simulink model "Control_Model"  (R2024b)
settings: Solver=FixedStepDiscrete  StartTime=0.0  StopTime=10.0  FixedStep=50e-6  MaxStep=1e-6  RelTol=1e-3
values from neighbouring files (symbols this model uses):
  Id_ki = Rs / tau    (= 1250)    [PID_Data.m]    (also in PMSM_PID_Data.m = 900)
  Id_kp = Ld / tau    (= 12.5)    [PID_Data.m]    (also in PMSM_PID_Data.m = 0.5)
  Iq_ki = Rs / tau    (= 1250)    [PID_Data.m]    (also in PMSM_PID_Data.m = 900)
  Iq_kp = Lq / tau    (= 12.5)    [PID_Data.m]    (also in PMSM_PID_Data.m = 0.5)
  Lambda = 0.175    [PID_Data.m]    (also in PMSM_PID_Data.m = (Ke_LL/sqrt(3)) / (p * 1000*2*pi/60))
  Ld = 0.005    [PID_Data.m]    (also in PMSM_PID_Data.m = 0.0002)
  lower_limit = -86.55    [PID_Data.m]    (also in PMSM_PID_Data.m = -20)
  Lq = 0.005    [PID_Data.m]    (also in PMSM_PID_Data.m = 0.0002)
  p = 4    [PID_Data.m]    (also in PMSM_PID_Data.m)
  Spd_Kb = Ki_radps    (= 47.619047619)    [PID_Data.m]    (also in PMSM_PID_Data.m = Spd_ki/Spd_kp)
  Spd_ki = Ki_radps*(2*pi/60)    (= 4.9866550057)    [PID_Data.m]    (also in PMSM_PID_Data.m = Ki_radps*(2*pi/60))
  Spd_kp = Kp_radps*(2*pi/60)    (= 0.0282045207122)    [PID_Data.m]    (also in PMSM_PID_Data.m = Kp_radps*(2*pi/60))
  Spd_lower_limit = -Iq_ref_limit    (= -10)    [PID_Data.m]    (also in PMSM_PID_Data.m = -7.1)
  Spd_upper_limit = Iq_ref_limit    (= 10)    [PID_Data.m]    (also in PMSM_PID_Data.m = 7.1)
  Ts = 1/20000    (= 5e-05)    [PID_Data.m]    (also in PMSM_PID_Data.m)
  Uabc_limit = 2/Vdc    (= 0.00666666666667)    [PID_Data.m]    (also in PMSM_PID_Data.m = 0.05)
  upper_limit = 86.55    [PID_Data.m]    (also in PMSM_PID_Data.m = 20)
  Vdc = 300    [PID_Data.m]    (also in PMSM_PID_Data.m = 40)
libraries: slpidlib x3, mcbcontrolslib x1
settings Model: Creator=BitCore  LastModifiedBy=BitCore

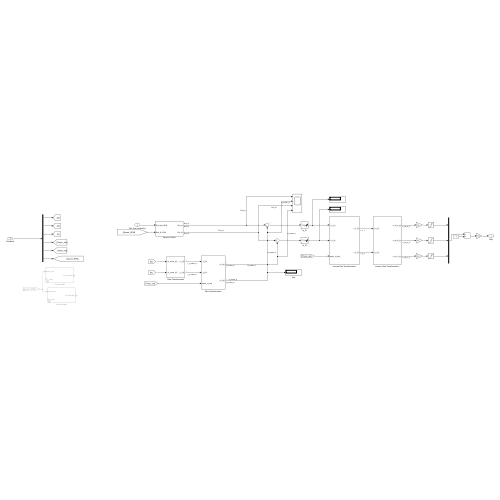
[thumbnail: Simulink's stored preview of the top-level diagram]
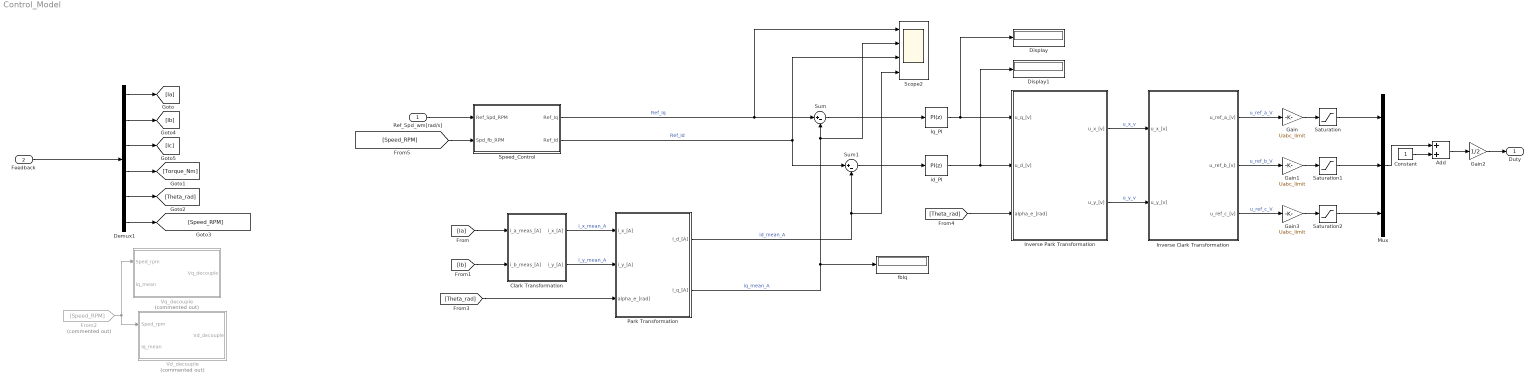
== system Control_Model ==
  Ref_Spd_wm[rad/s] : Inport
  Feedback : Inport  Port=2  OutDataTypeStr=single
  Add : Sum
  Clark Transformation : Subsystem
  Constant : Constant
  Demux1 : Demux  Outputs=6
  Display : Display
  Display1 : Display
  From2 : From  Commented=on  GotoTag=Speed_RPM
  Gain : Gain  Gain=Uabc_limit
  Gain1 : Gain  Gain=Uabc_limit
  Gain2 : Gain  Gain=1/2
  Gain3 : Gain  Gain=Uabc_limit
  "Inverse Clark Transformation " : Subsystem
  Inverse Park Transformation : Subsystem
  Iq_PI : slpidlib/PID Controller  Controller=PI  Form=Parallel  TimeDomain=Discrete-time  UseExternalTs=off  SampleTime=Ts  IntegratorMethod=Forward Euler  FilterMethod=Forward Euler  ControllerParametersSource=internal  P=Iq_kp  I=Iq_ki  UseKiTs=off  D=0  UseExternalDerivativeSource=off  N=100  UseFilter=on  TunerSelectOption=Transfer Function Based (PID Tuner App)  InitialConditionSource=internal  InitialConditionForIntegrator=0  InitialConditionForFilter=0  DifferentiatorICPrevScaledInput=0  ExternalReset=none  TrackingMode=off  Kt=1  LimitOutput=on  SatLimitsSource=internal  UpperSaturationLimit=upper_limit  LowerSaturationLimit=lower_limit  LinearizeAsGain=on  AntiWindupMode=back-calculation  Kb=1  LimitIntegrator=off  UpperIntegratorSaturationLimit=inf  LowerIntegratorSaturationLimit=-inf  POutMin=[]  POutMax=[]  IOutMin=[]  IOutMax=[]  DOutMin=[]  DOutMax=[]  NOutMin=[]  NOutMax=[]  SumOutMin=[]  SumOutMax=[]  SaturationOutMin=[]  SaturationOutMax=[]  PParamMin=[]  PParamMax=[]  IParamMin=[]  IParamMax=[]  DParamMin=[]  DParamMax=[]  NParamMin=[]  NParamMax=[]  KbParamMin=[]  KbParamMax=[]  KtParamMin=[]  KtParamMax=[]  KbOutMin=[]  KbOutMax=[]  KtOutMin=[]  KtOutMax=[]  IntegratorOutMin=[]  IntegratorOutMax=[]  FilterOutMin=[]  FilterOutMax=[]  SumI1OutMin=[]  SumI1OutMax=[]  SumI2OutMin=[]  SumI2OutMax=[]  SumI3OutMin=[]  SumI3OutMax=[]  SumI4OutMin=[]  SumI4OutMax=[]  SumDOutMin=[]  SumDOutMax=[]  DifferentiatorOutMin=[]  DifferentiatorOutMax=[]  FilterDiffOutCoefMin=[]  FilterDiffOutCoefMax=[]  ReciprocalOutMin=[]  ReciprocalOutMax=[]  SumDenOutMin=[]  SumDenOutMax=[]  SumNumOutMin=[]  SumNumOutMax=[]  DivideOutMin=[]  DivideOutMax=[]  UdiffTsProdOutMin=[]  UdiffTsProdOutMax=[]  NTsProdOutMin=[]  NTsProdOutMax=[]  UintegralTsProdOutMin=[]  UintegralTsProdOutMax=[]  UngainTsProdOutMin=[]  UngainTsProdOutMax=[]  ClampingZeroOutDataTypeStr=Inherit: Inherit via back propagation  ClampingZeroOutMin=[]  ClampingZeroOutMax=[]  FilterDenConstantOutDataTypeStr=Inherit: Inherit via back propagation  FilterDenConstantOutMin=[]  FilterDenConstantOutMax=[]  PCopyOutDataTypeStr=Inherit: Inherit via back propagation  PCopyOutMin=[]  PCopyOutMax=[]  NCopyOutDataTypeStr=Inherit: Inherit via back propagation  NCopyOutMin=[]  NCopyOutMax=[]  IntegratorContinuousStateAttributes=''  IntegratorStateMustResolveToSignalObject=off  IntegratorRTWStateStorageClass=Auto  FilterContinuousStateAttributes=''  FilterStateMustResolveToSignalObject=off  FilterRTWStateStorageClass=Auto  ParallelPVariant=InternalParameters  IdealPVariant=Disabled  IVariant=InternalParameters  DVariant=Disabled  IntegratorVariant=Discrete  SatVariant=Enabled  AWVariant=BackCalculation  PCopyVariant=Disabled  TRVariant=Disabled  FdbkBlocksVariant=Forward  IdealPFdbkVariant=Disabled  SatFdbkVariant=Disabled  DerivativeFilterVariant=Disabled  NVariant=Disabled  NCopyVariant=Disabled_SignalSpec  FilterICVariant=Disabled  IntegratorICVariant=InternalICs  ExternalResetVariant=Disabled  TRSumVariant=Passthrough  SumFdbkVariant=Disabled  SumVariant=Sum_PI  TsampFilterVariant=InternalTs  TsampNgainVariant=Passthrough  TsampIntegralVariant=Disabled_SignalSpec  ExternalSaturationOutDataTypeStr=Inherit: Same as second input  DerivativeSourceVariant=Disabled  PreIntVariant=InternalPreInt
  Mux : Mux  Inputs=3
  Park Transformation : Subsystem
  Saturation : Saturate  UpperLimit=1  LowerLimit=-1
  Saturation1 : Saturate  UpperLimit=1  LowerLimit=-1
  Saturation2 : Saturate  UpperLimit=1  LowerLimit=-1
  Scope2 : Scope  NumInputPorts=4
  Speed_Control : Subsystem
  Sum : Sum  Inputs=|+-
  Sum1 : Sum  Inputs=|+-
  Vd_decouple : Subsystem  Commented=on
  Vq_decouple : Subsystem  Commented=on
  fbIq : Display
  id_PI : slpidlib/PID Controller  Controller=PI  Form=Parallel  TimeDomain=Discrete-time  UseExternalTs=off  SampleTime=Ts  IntegratorMethod=Forward Euler  FilterMethod=Forward Euler  ControllerParametersSource=internal  P=Id_kp  I=Id_ki  UseKiTs=off  D=0  UseExternalDerivativeSource=off  N=100  UseFilter=on  TunerSelectOption=Transfer Function Based (PID Tuner App)  InitialConditionSource=internal  InitialConditionForIntegrator=0  InitialConditionForFilter=0  DifferentiatorICPrevScaledInput=0  ExternalReset=none  TrackingMode=off  Kt=1  LimitOutput=on  SatLimitsSource=internal  UpperSaturationLimit=upper_limit  LowerSaturationLimit=lower_limit  LinearizeAsGain=on  AntiWindupMode=back-calculation  Kb=1  LimitIntegrator=off  UpperIntegratorSaturationLimit=inf  LowerIntegratorSaturationLimit=-inf  POutMin=[]  POutMax=[]  IOutMin=[]  IOutMax=[]  DOutMin=[]  DOutMax=[]  NOutMin=[]  NOutMax=[]  SumOutMin=[]  SumOutMax=[]  SaturationOutMin=[]  SaturationOutMax=[]  PParamMin=[]  PParamMax=[]  IParamMin=[]  IParamMax=[]  DParamMin=[]  DParamMax=[]  NParamMin=[]  NParamMax=[]  KbParamMin=[]  KbParamMax=[]  KtParamMin=[]  KtParamMax=[]  KbOutMin=[]  KbOutMax=[]  KtOutMin=[]  KtOutMax=[]  IntegratorOutMin=[]  IntegratorOutMax=[]  FilterOutMin=[]  FilterOutMax=[]  SumI1OutMin=[]  SumI1OutMax=[]  SumI2OutMin=[]  SumI2OutMax=[]  SumI3OutMin=[]  SumI3OutMax=[]  SumI4OutMin=[]  SumI4OutMax=[]  SumDOutMin=[]  SumDOutMax=[]  DifferentiatorOutMin=[]  DifferentiatorOutMax=[]  FilterDiffOutCoefMin=[]  FilterDiffOutCoefMax=[]  ReciprocalOutMin=[]  ReciprocalOutMax=[]  SumDenOutMin=[]  SumDenOutMax=[]  SumNumOutMin=[]  SumNumOutMax=[]  DivideOutMin=[]  DivideOutMax=[]  UdiffTsProdOutMin=[]  UdiffTsProdOutMax=[]  NTsProdOutMin=[]  NTsProdOutMax=[]  UintegralTsProdOutMin=[]  UintegralTsProdOutMax=[]  UngainTsProdOutMin=[]  UngainTsProdOutMax=[]  ClampingZeroOutDataTypeStr=Inherit: Inherit via back propagation  ClampingZeroOutMin=[]  ClampingZeroOutMax=[]  FilterDenConstantOutDataTypeStr=Inherit: Inherit via back propagation  FilterDenConstantOutMin=[]  FilterDenConstantOutMax=[]  PCopyOutDataTypeStr=Inherit: Inherit via back propagation  PCopyOutMin=[]  PCopyOutMax=[]  NCopyOutDataTypeStr=Inherit: Inherit via back propagation  NCopyOutMin=[]  NCopyOutMax=[]  IntegratorContinuousStateAttributes=''  IntegratorStateMustResolveToSignalObject=off  IntegratorRTWStateStorageClass=Auto  FilterContinuousStateAttributes=''  FilterStateMustResolveToSignalObject=off  FilterRTWStateStorageClass=Auto  ParallelPVariant=InternalParameters  IdealPVariant=Disabled  IVariant=InternalParameters  DVariant=Disabled  IntegratorVariant=Discrete  SatVariant=Enabled  AWVariant=BackCalculation  PCopyVariant=Disabled  TRVariant=Disabled  FdbkBlocksVariant=Forward  IdealPFdbkVariant=Disabled  SatFdbkVariant=Disabled  DerivativeFilterVariant=Disabled  NVariant=Disabled  NCopyVariant=Disabled_SignalSpec  FilterICVariant=Disabled  IntegratorICVariant=InternalICs  ExternalResetVariant=Disabled  TRSumVariant=Passthrough  SumFdbkVariant=Disabled  SumVariant=Sum_PI  TsampFilterVariant=InternalTs  TsampNgainVariant=Passthrough  TsampIntegralVariant=Disabled_SignalSpec  ExternalSaturationOutDataTypeStr=Inherit: Same as second input  DerivativeSourceVariant=Disabled  PreIntVariant=InternalPreInt
  Duty : Outport
  wires:
  Feedback/1 -> Demux1/1
  Demux1/1 -> [Ia]
  Demux1/2 -> [Ib]
  Demux1/3 -> [Ic]
  Demux1/4 -> [Torque_Nm]
  Demux1/5 -> [Theta_rad]
  Demux1/6 -> [Speed_RPM]
  [Speed_RPM] -> Speed_Control/2(Spd_fb_RPM)
  Clark Transformation/1(i_x_[A]) -> Park Transformation/1(i_x_[A])  "i_x_mean_A"
  [Ib] -> Clark Transformation/2(i_b_meas_[A])
  [Ia] -> Clark Transformation/1(i_a_meas_[A])
  [Theta_rad] -> Park Transformation/3(alpha_e_[rad])
  Clark Transformation/2(i_y_[A]) -> Park Transformation/2(i_y_[A])  "i_y_mean_A"
  Sum/1 -> Iq_PI/1
  Sum1/1 -> id_PI/1
  [Theta_rad] -> Inverse Park Transformation/3(alpha_e_[rad])
  Inverse Park Transformation/1(u_x_[v]) -> "Inverse Clark Transformation "/1(u_x_[v])  "u_x_v"
  Inverse Park Transformation/2(u_y_[v]) -> "Inverse Clark Transformation "/2(u_y_[v])  "u_y_v"
  Ref_Spd_wm[rad/s]/1 -> Speed_Control/1(Ref_Spd_RPM)
  Park Transformation/1(I_d_[A]) -> Sum1/2, Scope2/4  "id_mean_A"
  Park Transformation/2(I_q_[A]) -> Scope2/2, Sum/2, fbIq/1  "iq_mean_A"
  "Inverse Clark Transformation "/1(u_ref_a_[v]) -> Gain/1  "u_ref_a_V"
  "Inverse Clark Transformation "/2(u_ref_b_[v]) -> Gain1/1  "u_ref_b_V"
  "Inverse Clark Transformation "/3(u_ref_c_[v]) -> Gain3/1  "u_ref_c_V"
  Gain/1 -> Saturation/1
  Gain1/1 -> Saturation1/1
  Saturation2/1 -> Mux/3
  Gain3/1 -> Saturation2/1
  Saturation/1 -> Mux/1
  Saturation1/1 -> Mux/2
  Mux/1 -> Add/1
  Constant/1 -> Add/2
  Add/1 -> Gain2/1
  Gain2/1 -> Duty/1
  From2/1 -> Vq_decouple/1(Sped_rpm), Vd_decouple/1(Sped_rpm)
  Iq_PI/1 -> Inverse Park Transformation/1(u_q_[v]), Display/1
  id_PI/1 -> Inverse Park Transformation/2(u_d_[v]), Display1/1
  Speed_Control/1(Ref_Iq) -> Scope2/1, Sum/1  "Ref_Iq"
  Speed_Control/2(Ref_Id) -> Scope2/3, Sum1/1  "Ref_Id"

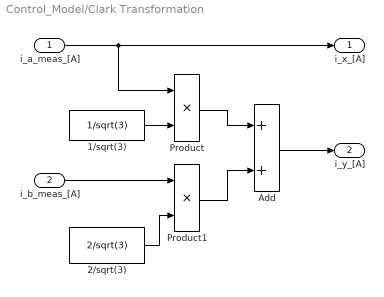
== system Control_Model/Clark Transformation ==
  i_a_meas_[A] : Inport
  i_b_meas_[A] : Inport  Port=2
  1/sqrt(3) : Constant  Value=1/sqrt(3)  OutDataTypeStr=single
  2/sqrt(3) : Constant  Value=2/sqrt(3)  OutDataTypeStr=single
  Add : Sum
  Product : Product
  Product1 : Product
  i_x_[A] : Outport
  i_y_[A] : Outport  Port=2
  wires:
  1/sqrt(3)/1 -> Product/2
  i_a_meas_[A]/1 -> Product/1, i_x_[A]/1
  i_b_meas_[A]/1 -> Product1/1
  2/sqrt(3)/1 -> Product1/2
  Product/1 -> Add/1
  Product1/1 -> Add/2
  Add/1 -> i_y_[A]/1

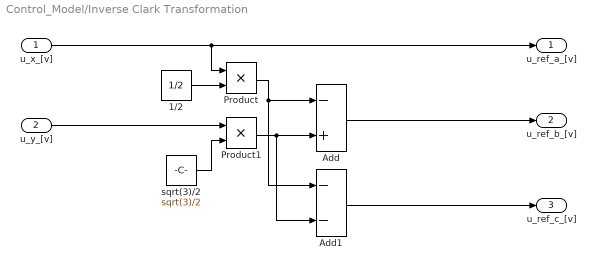
== system Control_Model/Inverse Clark Transformation  ==
  u_x_[v] : Inport
  u_y_[v] : Inport  Port=2
  1/2 : Constant  Value=1/2
  Add : Sum  Inputs=-+
  Add1 : Sum  Inputs=--
  Product : Product
  Product1 : Product
  sqrt(3)/2 : Constant  Value=sqrt(3)/2
  u_ref_a_[v] : Outport
  u_ref_b_[v] : Outport  Port=2
  u_ref_c_[v] : Outport  Port=3
  wires:
  u_x_[v]/1 -> Product/1, u_ref_a_[v]/1
  1/2/1 -> Product/2
  Product/1 -> Add1/1, Add/1
  u_y_[v]/1 -> Product1/1
  sqrt(3)/2/1 -> Product1/2
  Add/1 -> u_ref_b_[v]/1
  Product1/1 -> Add1/2, Add/2
  Add1/1 -> u_ref_c_[v]/1

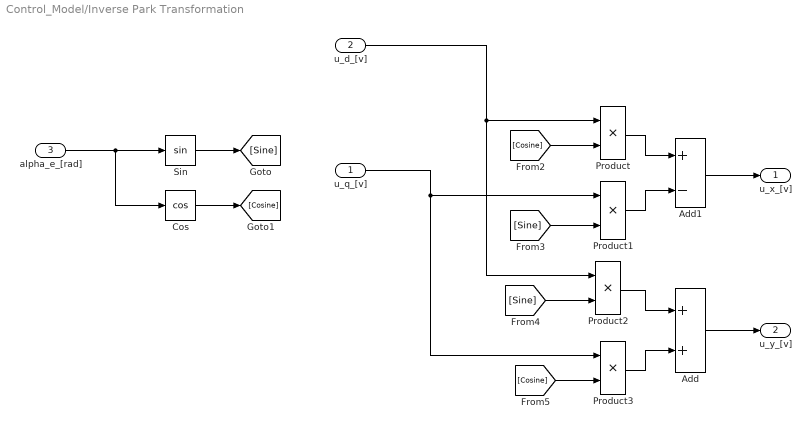
== system Control_Model/Inverse Park Transformation ==
  u_q_[v] : Inport
  u_d_[v] : Inport  Port=2
  alpha_e_[rad] : Inport  Port=3
  Add : Sum
  Add1 : Sum  Inputs=+-
  Cos : Trigonometry  Operator=cos
  Product{,1..3} (4 alike) : Product
  Sin : Trigonometry
  u_x_[v] : Outport
  u_y_[v] : Outport  Port=2
  wires:
  alpha_e_[rad]/1 -> Cos/1, Sin/1
  Sin/1 -> [Sine]
  Cos/1 -> [Cosine]
  u_d_[v]/1 -> Product2/1, Product/1
  [Cosine] -> Product/2
  u_q_[v]/1 -> Product3/1, Product1/1
  [Sine] -> Product1/2
  [Sine] -> Product2/2
  [Cosine] -> Product3/2
  Product2/1 -> Add/1
  Product3/1 -> Add/2
  Product1/1 -> Add1/2
  Product/1 -> Add1/1
  Add/1 -> u_y_[v]/1
  Add1/1 -> u_x_[v]/1

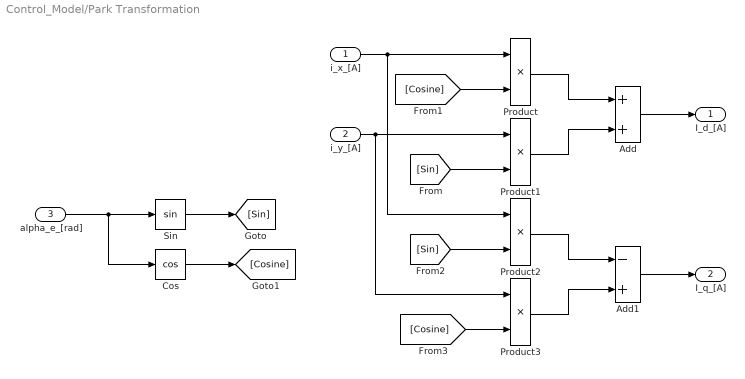
== system Control_Model/Park Transformation ==
  i_x_[A] : Inport
  i_y_[A] : Inport  Port=2
  alpha_e_[rad] : Inport  Port=3
  Add : Sum
  Add1 : Sum  Inputs=-+  AccumDataTypeStr=double
  Cos : Trigonometry  Operator=cos
  Product : Product
  Product1 : Product
  Product2 : Product  OutDataTypeStr=double
  Product3 : Product  OutDataTypeStr=double
  Sin : Trigonometry
  I_d_[A] : Outport
  I_q_[A] : Outport  Port=2
  wires:
  alpha_e_[rad]/1 -> Cos/1, Sin/1
  Sin/1 -> [Sin]
  Cos/1 -> [Cosine]
  i_x_[A]/1 -> Product2/1, Product/1
  [Cosine] -> Product/2
  [Sin] -> Product1/2
  [Sin] -> Product2/2
  [Cosine] -> Product3/2
  i_y_[A]/1 -> Product3/1, Product1/1
  Product/1 -> Add/1
  Product1/1 -> Add/2
  Product2/1 -> Add1/1
  Product3/1 -> Add1/2
  Add/1 -> I_d_[A]/1
  Add1/1 -> I_q_[A]/1

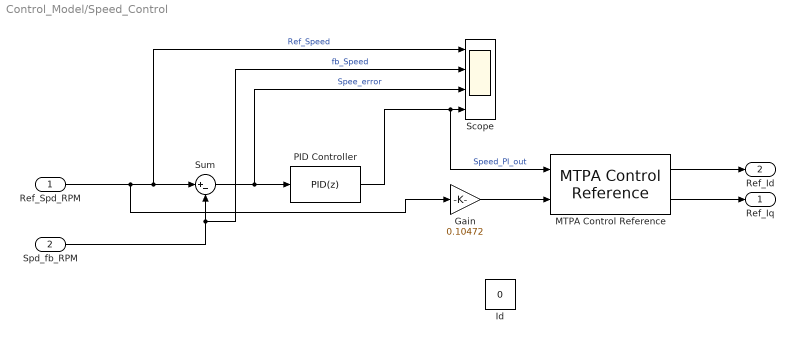
== system Control_Model/Speed_Control ==
  Ref_Spd_RPM : Inport
  Spd_fb_RPM : Inport  Port=2
  Gain : Gain  Gain=0.10472
  Id : Constant  Value=0
  MTPA Control Reference : mcbcontrolslib/MTPA Control Reference  VariantSelect=Surface PMSM  polePairs=p  Rs=0.36  Ld=Ld  Lq=0.4e-3  FluxPM=Lambda  ilimit=100  Vdc_input_select=Specify via dialog  V_dc=300  Units=Per-Unit (PU)  N_base=20000  I_base=19.3  T_base=0.74059  V_base=Vdc/sqrt(3)  N_base_disp=3182  MTPAiterator=on  iterCount=10
      settings: LibrarySourceBlock=mcblib/Controls/Control Reference/MTPA Control Reference
  PID Controller : slpidlib/PID Controller  Controller=PID  Form=Parallel  TimeDomain=Discrete-time  UseExternalTs=off  SampleTime=-1  IntegratorMethod=Forward Euler  FilterMethod=Forward Euler  ControllerParametersSource=internal  P=Spd_kp  I=Spd_ki  UseKiTs=off  D=0  UseExternalDerivativeSource=off  N=100  UseFilter=on  TunerSelectOption=Transfer Function Based (PID Tuner App)  InitialConditionSource=internal  InitialConditionForIntegrator=0  InitialConditionForFilter=0  DifferentiatorICPrevScaledInput=0  ExternalReset=none  TrackingMode=off  Kt=1  LimitOutput=on  SatLimitsSource=internal  UpperSaturationLimit=Spd_upper_limit  LowerSaturationLimit=Spd_lower_limit  LinearizeAsGain=on  AntiWindupMode=back-calculation  Kb=Spd_Kb  LimitIntegrator=off  UpperIntegratorSaturationLimit=inf  LowerIntegratorSaturationLimit=-inf  POutMin=[]  POutMax=[]  IOutMin=[]  IOutMax=[]  DOutMin=[]  DOutMax=[]  NOutMin=[]  NOutMax=[]  SumOutMin=[]  SumOutMax=[]  SaturationOutMin=[]  SaturationOutMax=[]  PParamMin=[]  PParamMax=[]  IParamMin=[]  IParamMax=[]  DParamMin=[]  DParamMax=[]  NParamMin=[]  NParamMax=[]  KbParamMin=[]  KbParamMax=[]  KtParamMin=[]  KtParamMax=[]  KbOutMin=[]  KbOutMax=[]  KtOutMin=[]  KtOutMax=[]  IntegratorOutMin=[]  IntegratorOutMax=[]  FilterOutMin=[]  FilterOutMax=[]  SumI1OutMin=[]  SumI1OutMax=[]  SumI2OutMin=[]  SumI2OutMax=[]  SumI3OutMin=[]  SumI3OutMax=[]  SumI4OutMin=[]  SumI4OutMax=[]  SumDOutMin=[]  SumDOutMax=[]  DifferentiatorOutMin=[]  DifferentiatorOutMax=[]  FilterDiffOutCoefMin=[]  FilterDiffOutCoefMax=[]  ReciprocalOutMin=[]  ReciprocalOutMax=[]  SumDenOutMin=[]  SumDenOutMax=[]  SumNumOutMin=[]  SumNumOutMax=[]  DivideOutMin=[]  DivideOutMax=[]  UdiffTsProdOutMin=[]  UdiffTsProdOutMax=[]  NTsProdOutMin=[]  NTsProdOutMax=[]  UintegralTsProdOutMin=[]  UintegralTsProdOutMax=[]  UngainTsProdOutMin=[]  UngainTsProdOutMax=[]  ClampingZeroOutDataTypeStr=Inherit: Inherit via back propagation  ClampingZeroOutMin=[]  ClampingZeroOutMax=[]  FilterDenConstantOutDataTypeStr=Inherit: Inherit via back propagation  FilterDenConstantOutMin=[]  FilterDenConstantOutMax=[]  PCopyOutDataTypeStr=Inherit: Inherit via back propagation  PCopyOutMin=[]  PCopyOutMax=[]  NCopyOutDataTypeStr=Inherit: Inherit via back propagation  NCopyOutMin=[]  NCopyOutMax=[]  IntegratorContinuousStateAttributes=''  IntegratorStateMustResolveToSignalObject=off  IntegratorRTWStateStorageClass=Auto  FilterContinuousStateAttributes=''  FilterStateMustResolveToSignalObject=off  FilterRTWStateStorageClass=Auto  ParallelPVariant=InternalParameters  IdealPVariant=Disabled  IVariant=InternalParameters  DVariant=InternalParameters  IntegratorVariant=Discrete  SatVariant=Enabled  AWVariant=BackCalculation  PCopyVariant=Disabled  TRVariant=Disabled  FdbkBlocksVariant=Forward  IdealPFdbkVariant=Disabled  SatFdbkVariant=Disabled  DerivativeFilterVariant=ForwardEulerFilter  NVariant=InternalParameters  NCopyVariant=Disabled  FilterICVariant=InternalICsFilter  IntegratorICVariant=InternalICs  ExternalResetVariant=Disabled  TRSumVariant=Passthrough  SumFdbkVariant=Disabled  SumVariant=Sum_PID  TsampFilterVariant=InternalTs  TsampNgainVariant=Passthrough  TsampIntegralVariant=Disabled_SignalSpec  ExternalSaturationOutDataTypeStr=Inherit: Same as second input  DerivativeSourceVariant=ErrorSignal  PreIntVariant=InternalPreInt
  Scope : Scope  NumInputPorts=4
  Sum : Sum  Inputs=|+-
  Ref_Iq : Outport
  Ref_Id : Outport  Port=2
  wires:
  Sum/1 -> Scope/3, PID Controller/1  "Spee_error"
  PID Controller/1 -> MTPA Control Reference/1, Scope/4  "Speed_PI_out"
  Ref_Spd_RPM/1 -> Gain/1, Scope/1, Sum/1  "Ref_Speed"
  Spd_fb_RPM/1 -> Scope/2, Sum/2  "fb_Speed"
  MTPA Control Reference/2 -> Ref_Iq/1
  MTPA Control Reference/1 -> Ref_Id/1
  Gain/1 -> MTPA Control Reference/2

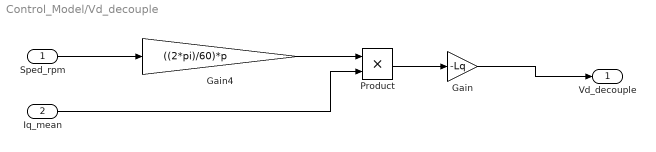
== system Control_Model/Vd_decouple ==
  Sped_rpm : Inport
  Iq_mean : Inport  Port=2
  Gain : Gain  Gain=-Lq
  Gain4 : Gain  Gain=((2*pi)/60)*p
  Product : Product
  Vd_decouple : Outport
  wires:
  Product/1 -> Gain/1
  Iq_mean/1 -> Product/2
  Gain4/1 -> Product/1
  Sped_rpm/1 -> Gain4/1
  Gain/1 -> Vd_decouple/1

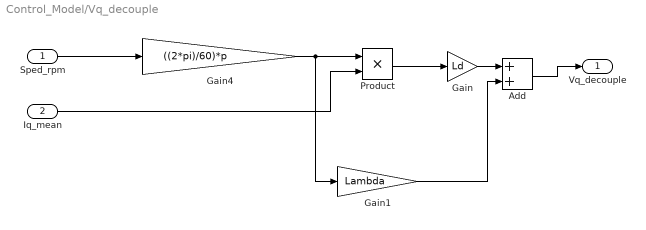
== system Control_Model/Vq_decouple ==
  Sped_rpm : Inport
  Iq_mean : Inport  Port=2
  Add : Sum
  Gain : Gain  Gain=Ld
  Gain1 : Gain  Gain=Lambda
  Gain4 : Gain  Gain=((2*pi)/60)*p
  Product : Product
  Vq_decouple : Outport
  wires:
  Sped_rpm/1 -> Gain4/1
  Gain4/1 -> Gain1/1, Product/1
  Iq_mean/1 -> Product/2
  Product/1 -> Gain/1
  Gain/1 -> Add/1
  Add/1 -> Vq_decouple/1
  Gain1/1 -> Add/2
